simulink model "a2_pfc_rl"  (R2021b)
settings: Solver=FixedStepAuto  StartTime=0.0  StopTime=120  FixedStep=0.2  RelTol=1e-3
PreLoadFcn:
  | % Simulation parameters
  | %load exampleMap
InitFcn:
  | % paremeters of pure persuit
  | desired_v_robot_1=0.2
  | desired_w_robot_1=4
  | desired_lookahead_robot_1=0.2
  | 
  | % paremeters of recovery
  | recovery_w=0.5
  | 
  | sampleTime = 0.05;
  | 
  | % Robot parameters
  | wheelRadius = 0.025;
  | robotRadius = 0.15;
  | 
  | % Lidar parameters
  | sensorOffset = [0,0];
  | scanAngles = linspace(-pi/2,pi/2,9)';
  | maxRange = 5;
  | 
  | %%%%%%
  | ks=-1;
  | 
  | %初始位置
  | x_1_0=1;
  | y_1_0=0;
  | yaw_1_0=0.0;
  | 
  | x_2_0=0.6;
  | y_2_0=0;
  | yaw_2_0=0;
  | x_3_0=0;
  | y_3_0=0.6;
  | yaw_3_0=0;
  | 
  | x_4_0=0;
  | y_4_0=0.9;
  | yaw_4_0=0;
libraries: mobileRoboticsLib x3, simulink x2, robotmobilelib x2, robotalgslib x1, rllib x1
settings Model: Creator=scastro  LastModifiedBy=amov
settings SolverCC: ZeroCrossAlgorithm=Adaptive  AlgebraicLoopSolver=TrustRegion
settings DataIOCC: ReturnWorkspaceOutputs=off
settings OptimizationCC: EnhancedBackFolding=on  PassReuseOutputArgsAs=Individual arguments  ZeroExternalMemoryAtStartup=off  ZeroInternalMemoryAtStartup=off  MaxStackSize=64  OptimizeBlockOrder=speed  DifferentSizesBufferReuse=on  OptimizationCustomize=off  EfficientTunableParamExpr=on
settings DebuggingCC: ParameterTunabilityLossMsg=error  PregeneratedLibrarySubsystemCodeDiagnostic=none  SFMachineParentedDataDiag=warning  ArithmeticOperatorsInVariantConditions=warning
settings HardwareCC: ProdBitPerPointer=32  ProdBitPerSizeT=32  ProdBitPerPtrDiffT=32  ProdLargestAtomicFloat=None  ProdIntDivRoundTo=Undefined  ProdEndianess=Unspecified  ProdWordSize=32  ProdHWDeviceType=Generic->Unspecified (assume 32-bit Generic)
settings SFSimCC: SimUseLocalCustomCode=off  MATLABDynamicMemAlloc=off  CustomCodeUndefinedFunction=UseInterfaceOnly
settings RTWCC: Description=Embedded Coder  SystemTargetFile=ert.tlc  HardwareBoard=Robot Operating System (ROS)  TLCOptions="-aInlineSetEventsForThisBaseRateFcn=TLC_FALSE -aSuppressMultiTaskScheduler=TLC_FALSE  -aRateBasedStepFcn=0"  TemplateMakefile=ert_default_tmf  RTWUseLocalCustomCode=off  Toolchain=Catkin  TargetLang=C++
settings CodeAppCC: ForceParamTrailComments=on  IgnoreCustomStorageClasses=off  OperatorAnnotations=on  SimulinkDataObjDesc=on  SFDataObjDesc=on  InsertBlockDesc=on

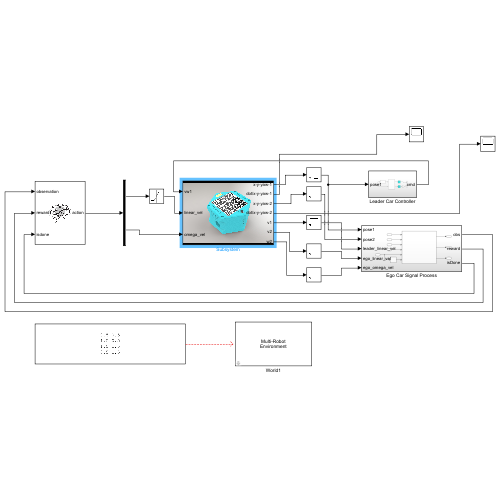
[thumbnail: Simulink's stored preview of the top-level diagram]
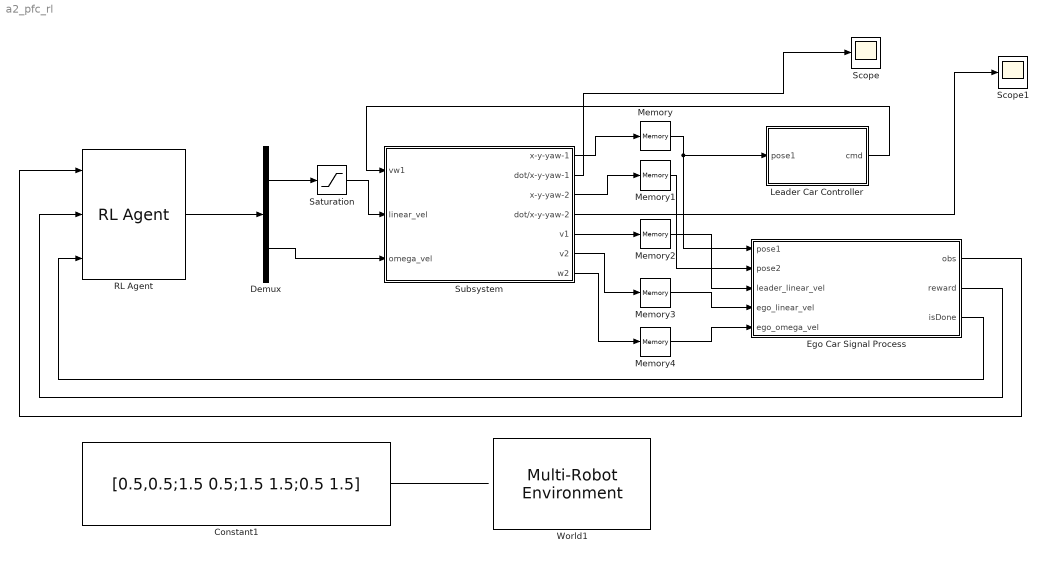
== system a2_pfc_rl ==
  Constant1 : Constant  Value=[0.5,0.5;1.5 0.5;1.5 1.5;0.5 1.5]
  Demux : Demux  Outputs=2
  Ego Car Signal Process : Subsystem
  Leader Car Controller : Subsystem
  Memory : Memory  InitialCondition=[x_1_0,y_1_0,yaw_1_0]
  Memory1 : Memory  InitialCondition=[x_2_0,y_2_0,yaw_2_0]
  Memory2 : Memory  InitialCondition=0.2
  Memory3 : Memory  InitialCondition=0.2
  Memory4 : Memory
  RL Agent : rllib/RL Agent  Agent=agent  ExternalActionAsInput=off  ProvideCumRwd=off  TreatAsDirectFeedthrough=on
  Saturation : Saturate  LowerLimit=0.1
  Scope : Scope
  Scope1 : Scope
  Subsystem : Subsystem
      mask Display: image('$imagefile'); % 使用工具条上的 "编辑图像" 进行更改。
  World1 : mobileRoboticsLib/Environments/Multi-Robot Environment  numRobots=2  showWaypoints=on  showObjects=off  objectColors=[1 0 0;0 1 0;0 0 1]  objectMarkers='s'  showRobotIds=on  plotSensorLines=on
      settings: SourceProductName=Mobile Robotics Simulation Toolbox
  wires:
  Subsystem/1(x-y-yaw-1) -> Memory/1
  Subsystem/3(x-y-yaw-2) -> Memory1/1
  Subsystem/5(v1) -> Memory2/1
  Subsystem/6(v2) -> Memory3/1
  Subsystem/7(w2) -> Memory4/1
  Memory1/1 -> Ego Car Signal Process/2(pose2)
  Memory2/1 -> Ego Car Signal Process/3(leader_linear_vel)
  Memory3/1 -> Ego Car Signal Process/4(ego_linear_vel)
  Memory4/1 -> Ego Car Signal Process/5(ego_omega_vel)
  Ego Car Signal Process/3(isDone) -> RL Agent/3
  Saturation/1 -> Subsystem/2(linear_vel)
  Demux/2 -> Subsystem/3(omega_vel)
  Subsystem/2(dot/x-y-yaw-1) -> Scope/1
  Subsystem/4(dot/x-y-yaw-2) -> Scope1/1
  Ego Car Signal Process/1(obs) -> RL Agent/1
  Ego Car Signal Process/2(reward) -> RL Agent/2
  RL Agent/1 -> Demux/1
  Demux/1 -> Saturation/1
  Memory/1 -> Ego Car Signal Process/1(pose1), Leader Car Controller/1(pose1)
  Leader Car Controller/1(cmd) -> Subsystem/1(vw1)
  Constant1/1 -> ?

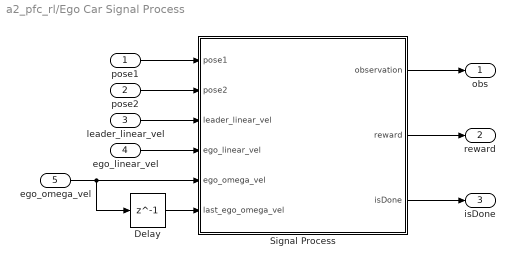
== system a2_pfc_rl/Ego Car Signal Process ==
  pose1 : Inport
  pose2 : Inport  Port=2
  leader_linear_vel : Inport  Port=3
  ego_linear_vel : Inport  Port=4
  ego_omega_vel : Inport  Port=5
  Delay : Delay  DelayLength=1  InitialCondition=0
  Signal Process : MATLAB Function  TreatAsAtomicUnit=on
  obs : Outport
  reward : Outport  Port=2
  isDone : Outport  Port=3
  wires:
  pose1/1 -> Signal Process/1(pose1)
  Signal Process/1(observation) -> obs/1
  leader_linear_vel/1 -> Signal Process/3(leader_linear_vel)
  Signal Process/3(isDone) -> isDone/1
  ego_omega_vel/1 -> Signal Process/5(ego_omega_vel), Delay/1
  pose2/1 -> Signal Process/2(pose2)
  ego_linear_vel/1 -> Signal Process/4(ego_linear_vel)
  Signal Process/2(reward) -> reward/1
  Delay/1 -> Signal Process/6(last_ego_omega_vel)

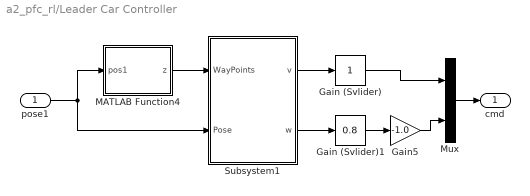
== system a2_pfc_rl/Leader Car Controller ==
  pose1 : Inport
  Gain (Svlider) : simulink/Math Operations/Slider Gain  gain=1  low=0.1  high=10
  Gain (Svlider)1 : simulink/Math Operations/Slider Gain  gain=0.8  low=0.1  high=3
  Gain5 : Gain  Gain=-1.0
  MATLAB Function4 : MATLAB Function  TreatAsAtomicUnit=on
  Mux : Mux  Inputs=2
  Subsystem1 : Subsystem
  cmd : Outport
  wires:
  Mux/1 -> cmd/1
  Subsystem1/1(v) -> Gain (Svlider)/1
  Gain (Svlider)/1 -> Mux/1
  pose1/1 -> Subsystem1/2(Pose), MATLAB Function4/1(pos1)
  Subsystem1/2(w) -> Gain (Svlider)1/1
  MATLAB Function4/1(z) -> Subsystem1/1(WayPoints)
  Gain (Svlider)1/1 -> Gain5/1
  Gain5/1 -> Mux/2

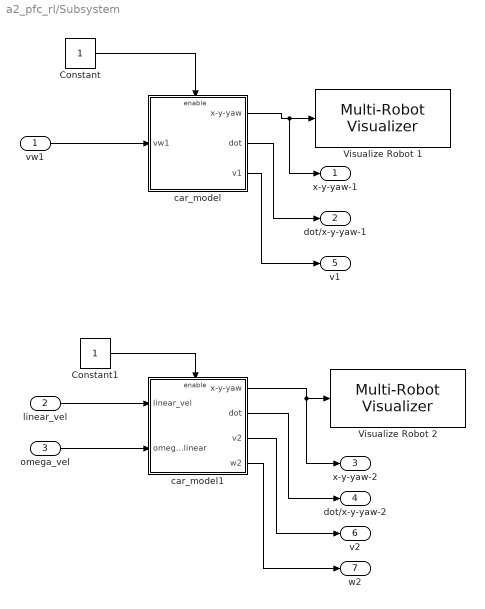
== system a2_pfc_rl/Subsystem ==
  vw1 : Inport
  linear_vel : Inport  Port=2
  omega_vel : Inport  Port=3
  Constant : Constant
  Constant1 : Constant
  Visualize Robot 1 : mobileRoboticsLib/Environments/Multi-Robot Visualizer  idx=1  radius=0.15  robotColor=[0 0 1]  showTraj=off  hasLidar=off  sensorOffset=sensorOffset  scanAngles=scanAngles  maxNumScans=0  hasObjDetector=off  objDetectorOffset=[0,0]  objDetectorAngle=0  objDetectorFOV=pi/2  objDetectorMaxRange=5  hasRobotDetector=off  robotDetectorOffset=[0,0]  robotDetectorAngle=0  robotDetectorFOV=pi/3  robotDetectorMaxRange=5  robotDetectorNumDetections=0
      settings: SourceProductName=Mobile Robotics Simulation Toolbox
  Visualize Robot 2 : mobileRoboticsLib/Environments/Multi-Robot Visualizer  idx=2  radius=0.15  robotColor=[1 0 0]  showTraj=on  hasLidar=off  sensorOffset=sensorOffset  scanAngles=scanAngles  maxNumScans=0  hasObjDetector=off  objDetectorOffset=[0 0]  objDetectorAngle=0  objDetectorFOV=pi/2  objDetectorMaxRange=5  hasRobotDetector=off  robotDetectorOffset=[0,0]  robotDetectorAngle=0  robotDetectorFOV=pi/3  robotDetectorMaxRange=5  robotDetectorNumDetections=0
      settings: SourceProductName=Mobile Robotics Simulation Toolbox
  car_model : Subsystem
  car_model1 : Subsystem
  x-y-yaw-1 : Outport
  dot/x-y-yaw-1 : Outport  Port=2
  x-y-yaw-2 : Outport  Port=3
  dot/x-y-yaw-2 : Outport  Port=4
  v1 : Outport  Port=5
  v2 : Outport  Port=6
  w2 : Outport  Port=7
  wires:
  Constant/1 -> car_model/Enable
  Constant1/1 -> car_model1/Enable
  car_model/1(x-y-yaw) -> x-y-yaw-1/1, Visualize Robot 1/1
  car_model1/1(x-y-yaw) -> x-y-yaw-2/1, Visualize Robot 2/1
  vw1/1 -> car_model/1(vw1)
  car_model/2(dot) -> dot/x-y-yaw-1/1
  car_model1/2(dot) -> dot/x-y-yaw-2/1
  car_model/3(v1) -> v1/1
  car_model1/3(v2) -> v2/1
  car_model1/4(w2) -> w2/1
  omega_vel/1 -> car_model1/2(omega_linear)
  linear_vel/1 -> car_model1/1(linear_vel)

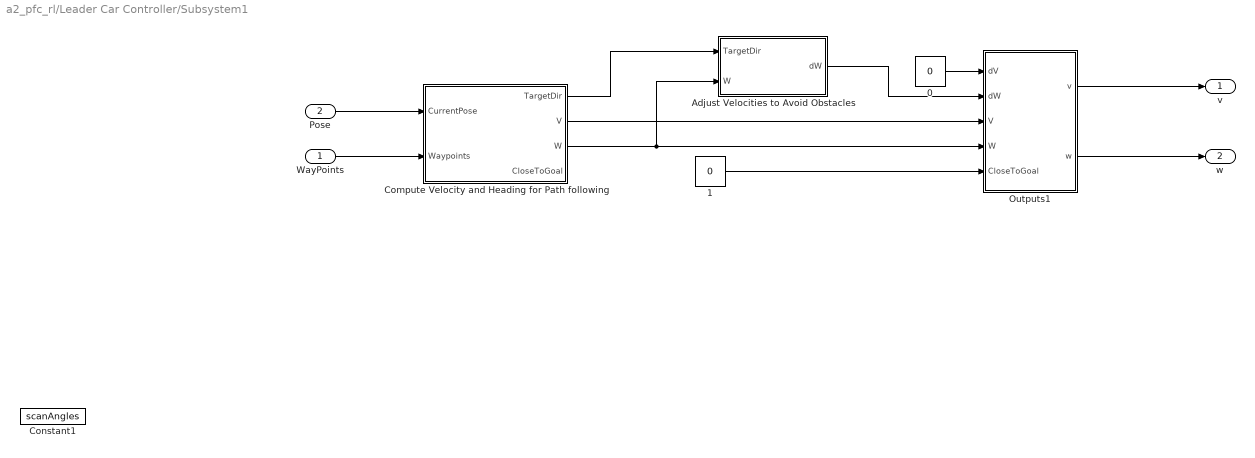
== system a2_pfc_rl/Leader Car Controller/Subsystem1 ==
  WayPoints : Inport
  Pose : Inport  Port=2
  0 : Constant  Value=0
  1 : Constant  Value=0
  Adjust Velocities to Avoid Obstacles : Subsystem
  Compute Velocity and Heading for Path following : Subsystem
  Constant1 : Constant  Value=scanAngles
  Outputs1 : Subsystem
  v : Outport
  w : Outport  Port=2
  wires:
  Compute Velocity and Heading for Path following/3(W) -> Adjust Velocities to Avoid Obstacles/2(W), Outputs1/4(W)
  Pose/1 -> Compute Velocity and Heading for Path following/1(CurrentPose)
  Compute Velocity and Heading for Path following/2(V) -> Outputs1/3(V)
  WayPoints/1 -> Compute Velocity and Heading for Path following/2(Waypoints)
  1/1 -> Outputs1/5(CloseToGoal)
  Outputs1/1(v) -> v/1
  Outputs1/2(w) -> w/1
  Adjust Velocities to Avoid Obstacles/1(dW) -> Outputs1/2(dW)
  0/1 -> Outputs1/1(dV)
  Compute Velocity and Heading for Path following/1(TargetDir) -> Adjust Velocities to Avoid Obstacles/1(TargetDir)

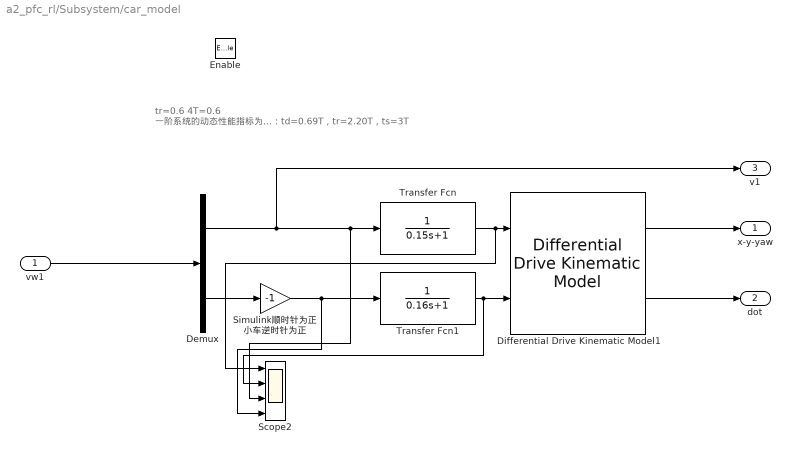
== system a2_pfc_rl/Subsystem/car_model ==
  note: tr=0.6
      | 4T=0.6
      | 一阶系统的动态性能指标为：td=0.69T，tr=2.20T，ts=3T
  vw1 : Inport
  Enable : EnablePort  ShowOutputPort=on
  Demux : Demux  Outputs=2
  Differential Drive Kinematic Model1 : robotmobilelib/Differential Drive Kinematic Model  VehicleInputs=Vehicle Speed & Heading Angular Velocity  WheelRadius=0.05  WheelSpeedRange=[-inf inf]  TrackWidth=0.2  InitialState=[x_1_0, y_1_0, yaw_1_0]'  SimulateUsing=Interpreted execution
      settings: SourceProductBaseCode=RO
  Scope2 : Scope  NumInputPorts=4
  Simulink顺时针为正 小车逆时针为正 : Gain  Gain=-1
  Transfer Fcn : TransferFcn  Denominator=[0.15 1]
  Transfer Fcn1 : TransferFcn  Denominator=[0.16 1]
  x-y-yaw : Outport
  dot : Outport  Port=2
  v1 : Outport  Port=3
  wires:
  Simulink顺时针为正 小车逆时针为正/1 -> Scope2/4, Transfer Fcn1/1
  Transfer Fcn/1 -> Differential Drive Kinematic Model1/1, Scope2/1
  Demux/1 -> Scope2/3, Transfer Fcn/1, v1/1
  Transfer Fcn1/1 -> Differential Drive Kinematic Model1/2, Scope2/2
  Demux/2 -> Simulink顺时针为正 小车逆时针为正/1
  vw1/1 -> Demux/1
  Differential Drive Kinematic Model1/1 -> x-y-yaw/1
  Differential Drive Kinematic Model1/2 -> dot/1

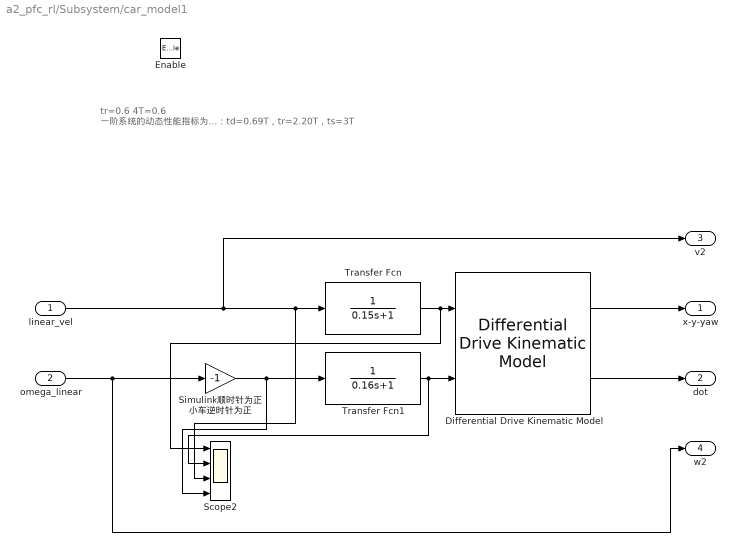
== system a2_pfc_rl/Subsystem/car_model1 ==
  note: tr=0.6
      | 4T=0.6
      | 一阶系统的动态性能指标为：td=0.69T，tr=2.20T，ts=3T
  linear_vel : Inport
  omega_linear : Inport  Port=2
  Enable : EnablePort  ShowOutputPort=on
  Differential Drive Kinematic Model : robotmobilelib/Differential Drive Kinematic Model  VehicleInputs=Vehicle Speed & Heading Angular Velocity  WheelRadius=0.05  WheelSpeedRange=[-inf inf]  TrackWidth=0.2  InitialState=[x_2_0, y_2_0, yaw_2_0]'  SimulateUsing=Interpreted execution
      settings: SourceProductBaseCode=RO
  Scope2 : Scope  NumInputPorts=4
  Simulink顺时针为正 小车逆时针为正 : Gain  Gain=-1
  Transfer Fcn : TransferFcn  Denominator=[0.15 1]
  Transfer Fcn1 : TransferFcn  Denominator=[0.16 1]
  x-y-yaw : Outport
  dot : Outport  Port=2
  v2 : Outport  Port=3
  w2 : Outport  Port=4
  wires:
  Simulink顺时针为正 小车逆时针为正/1 -> Scope2/4, Transfer Fcn1/1
  Transfer Fcn/1 -> Scope2/1, Differential Drive Kinematic Model/1
  linear_vel/1 -> v2/1, Scope2/3, Transfer Fcn/1
  Transfer Fcn1/1 -> Scope2/2, Differential Drive Kinematic Model/2
  Differential Drive Kinematic Model/1 -> x-y-yaw/1
  Differential Drive Kinematic Model/2 -> dot/1
  omega_linear/1 -> w2/1, Simulink顺时针为正 小车逆时针为正/1

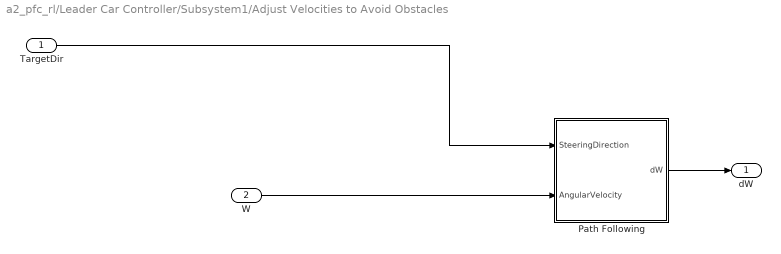
== system a2_pfc_rl/Leader Car Controller/Subsystem1/Adjust Velocities to Avoid Obstacles ==
  TargetDir : Inport
  W : Inport  Port=2
  Path Following : Subsystem  TreatAsAtomicUnit=on
  dW : Outport  VectorParamsAs1DForOutWhenUnconnected=off
  wires:
  Path Following/1(dW) -> dW/1
  W/1 -> Path Following/2(AngularVelocity)
  TargetDir/1 -> Path Following/1(SteeringDirection)

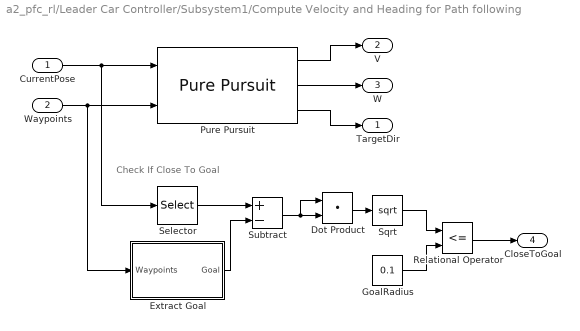
== system a2_pfc_rl/Leader Car Controller/Subsystem1/Compute Velocity and Heading for Path following ==
  note: Check If Close To Goal
  CurrentPose : Inport
  Waypoints : Inport  Port=2
  " Extract Goal" : MATLAB Function  TreatAsAtomicUnit=on
  Dot Product : DotProduct  InputSameDT=on  OutDataTypeStr=Inherit: Inherit via internal rule
  GoalRadius : Constant  Value=0.1
  Pure Pursuit : robotalgslib/Pure Pursuit  DesiredLinearVelocity=desired_v_robot_1  MaxAngularVelocity=desired_w_robot_1  LookaheadDistance=desired_lookahead_robot_1  TargetDirPort=on  SimulateUsing=Code generation
  Relational Operator : RelationalOperator  Operator=<=  OutDataTypeStr=boolean  RndMeth=Simplest
  Selector : Selector  InputPortWidth=3  IndexOptions=Index vector (dialog)  Indices=[1 2]  OutputSizes=1
  Sqrt : Sqrt  SaturateOnIntegerOverflow=on
  Subtract : Sum  Inputs=+-
  TargetDir : Outport  VectorParamsAs1DForOutWhenUnconnected=off
  V : Outport  Port=2  VectorParamsAs1DForOutWhenUnconnected=off
  W : Outport  Port=3  VectorParamsAs1DForOutWhenUnconnected=off
  CloseToGoal : Outport  Port=4  VectorParamsAs1DForOutWhenUnconnected=off
  wires:
  Pure Pursuit/3 -> TargetDir/1
  Pure Pursuit/2 -> W/1
  Pure Pursuit/1 -> V/1
  " Extract Goal"/1(Goal) -> Subtract/2
  Waypoints/1 -> " Extract Goal"/1(Waypoints), Pure Pursuit/2
  CurrentPose/1 -> Selector/1, Pure Pursuit/1
  Relational Operator/1 -> CloseToGoal/1
  GoalRadius/1 -> Relational Operator/2
  Selector/1 -> Subtract/1
  Dot Product/1 -> Sqrt/1
  Sqrt/1 -> Relational Operator/1
  Subtract/1 -> Dot Product/1, Dot Product/2

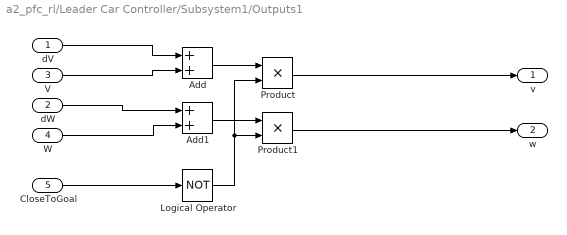
== system a2_pfc_rl/Leader Car Controller/Subsystem1/Outputs1 ==
  dV : Inport
  dW : Inport  Port=2
  V : Inport  Port=3
  W : Inport  Port=4
  CloseToGoal : Inport  Port=5
  Add : Sum
  Add1 : Sum
  Logical Operator : Logic  Operator=NOT  AllPortsSameDT=off  OutDataTypeStr=boolean
  Product : Product
  Product1 : Product
  v : Outport
  w : Outport  Port=2
  wires:
  V/1 -> Add/2
  W/1 -> Add1/2
  dV/1 -> Add/1
  dW/1 -> Add1/1
  CloseToGoal/1 -> Logical Operator/1
  Add/1 -> Product/1
  Add1/1 -> Product1/1
  Product1/1 -> w/1
  Product/1 -> v/1
  Logical Operator/1 -> Product1/2, Product/2

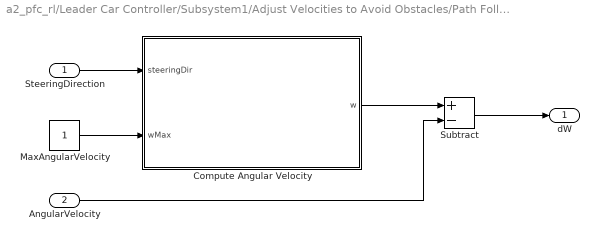
== system a2_pfc_rl/Leader Car Controller/Subsystem1/Adjust Velocities to Avoid Obstacles/Path Following ==
  SteeringDirection : Inport
  AngularVelocity : Inport  Port=2
  Compute Angular Velocity : MATLAB Function  TreatAsAtomicUnit=on
  MaxAngularVelocity : Constant
  Subtract : Sum  Inputs=+-
  dW : Outport  VectorParamsAs1DForOutWhenUnconnected=off
  wires:
  MaxAngularVelocity/1 -> Compute Angular Velocity/2(wMax)
  SteeringDirection/1 -> Compute Angular Velocity/1(steeringDir)
  Subtract/1 -> dW/1
  Compute Angular Velocity/1(w) -> Subtract/1
  AngularVelocity/1 -> Subtract/2

== matlab function a2_pfc_rl/Ego Car Signal Process/Signal Process ==
  data: observation output; reward output; isDone output; pose1 input; pose2 input; leader_linear_vel input size=1; ego_linear_vel input size=1; ego_omega_vel input size=1; last_ego_omega_vel input
function [observation, reward, isDone] = ...
    car2(pose1,pose2,leader_linear_vel, ego_linear_vel, ego_omega_vel, last_ego_omega_vel)


persistent sim_step  yaw_delta lateral_rel_dist

if isempty(sim_step)
    sim_step = 0;
end

if isempty(yaw_delta)
    yaw_delta = 0.0;
end

if isempty(lateral_rel_dist)
    lateral_rel_dist = 0.0;
end

x1=pose1(1);
y1=pose1(2);
yaw1=pose1(3);

x2=pose2(1);
y2=pose2(2);
yaw2=pose2(3);

observation = zeros(1,9);

isDone = 0;

yaw_delta_new = angdiff(yaw1, yaw2);

[rel_dist_new, lateral_rel_dist_new, longitudinal_rel_dist_new] = heng_zong_dist_calc(x1,y1,x2,y2, yaw1);

observation = get_obs(x1,x2,y1,y2,lateral_rel_dist_new, longitudinal_rel_dist_new, ...
    yaw_delta_new, leader_linear_vel, ego_linear_vel, yaw_delta, lateral_rel_dist);


isDone = EnvisDone(rel_dist_new, lateral_rel_dist_new, longitudinal_rel_dist_new);

e_v = observation(4);

reward = reward_calc(e_v, lateral_rel_dist_new, longitudinal_rel_dist_new, ego_linear_vel, ego_omega_vel, last_ego_omega_vel, isDone, sim_step);

sim_step = sim_step + 1;
yaw_delta = yaw_delta_new;
lateral_rel_dist = lateral_rel_dist_new;

end

function [rel_dist, heng_dist, zong_dist] = heng_zong_dist_calc(x1,y1,x2,y2, yaw1)

rel_yaw = atan2(y2-y1, x2-x1);

yaw_delta = angdiff(yaw1, rel_yaw);

rel_dist = sqrt(power(x2-x1,2.0)+power(y2-y1,2.0));

heng_dist = rel_dist*sin(yaw_delta);

zong_dist = rel_dist*cos(yaw_delta);

end

function v_ref = get_ref_velocity(leader_linear_vel, ego_linear_vel, longitudinal_rel_dist)
    t_gap = 1.0;
    D_default = 0.3;
    ego_v_set = 0.2;
    d_safe = ego_linear_vel * t_gap + D_default;

    if d_safe > longitudinal_rel_dist
        v_ref = min(leader_linear_vel, ego_v_set);
    else
        v_ref = ego_v_set;
    end
end

function observation = get_obs(x1,x2,y1,y2,lateral_rel_dist_new, longitudinal_rel_dist_new, ...
    yaw_delta_new, leader_linear_vel, ego_linear_vel, yaw_delta, lateral_rel_dist)  
    % 状态空间
    % longitudinal_rel_dist 前车与后车的纵向相对距离
    % lateral_rel_dist 前车与后车的横向相对距离
    % yaw_delta 前车与后车的航向角偏差
    % ego_linear_vel 后车的线速度
    % e_v 后车的参考速度与线速度之差
    % lateral_rel_dist_dot 前车与后车的横向相对距离变化率
    % yaw_delta_dot 前车与后车的航向角偏差变化率

    % 计算前车与后车的相对位置
    x_delta = x1 - x2;
    y_delta = y1 - y2;
    
    % 计算后车的横向偏移距离变化率和相对航向角变化率
    lateral_rel_dist_dot = lateral_rel_dist_new - lateral_rel_dist;
    yaw_delta_dot = yaw_delta_new - yaw_delta;

    % 计算后车的参考速度与线速度之差
    v_ref = get_ref_velocity(leader_linear_vel, ego_linear_vel, longitudinal_rel_dist_new);
    e_v = v_ref - ego_linear_vel;

    observation = [x_delta/2.0, y_delta/2.0, longitudinal_rel_dist_new/2.0, e_v/0.5, ego_linear_vel/0.5, ...
        lateral_rel_dist_new/2.0, lateral_rel_dist_dot/2.0, yaw_delta_new/pi, yaw_delta_dot/pi];
end

function flag = EnvisDone(rel_dist, lateral_rel_dist, longitudinal_rel_dist)
    flag = 0;
    avoid_dist = 0.18;

    max_lateral_rel_dist= 0.45;
    min_longitudinal_rel_dist = -0.5;

    if rel_dist <= avoid_dist
        flag = 1;
    end

    if longitudinal_rel_dist <= min_longitudinal_rel_dist || longitudinal_rel_dist >= 0
        flag = 1;
    end
    
    if abs(lateral_rel_dist) >= max_lateral_rel_dist
        flag = 1;
    end
end

function reward = reward_calc(e_v, lateral_rel_dist, longitudinal_rel_dist, ego_linear_vel, ego_omega_vel, last_ego_omega_vel, isDone, sim_step)
    F_t = 0.0;
    M_t = 0.0;
    H_t = 0.0;
    delta_omega = 0.0;
    
    e_v_square = e_v * e_v;
    lateral_rel_dist_square = lateral_rel_dist * lateral_rel_dist;
    longitudinal_rel_dist_square = longitudinal_rel_dist * longitudinal_rel_dist;

    if isDone==1
        F_t = 1.0;
    end

    if e_v_square < 1.0
        M_t = 1.0;
    end

    if lateral_rel_dist_square<0.01
        H_t = 1.0;
    end

    if sim_step >= 2
        delta_omega = ego_omega_vel - last_ego_omega_vel;
    end

    reward = -0.1*e_v_square - 0.1*ego_linear_vel*ego_linear_vel -0.3*lateral_rel_dist_square -0.3*longitudinal_rel_dist_square...
         - 0.5*ego_omega_vel*ego_omega_vel -0.4*delta_omega*delta_omega - 10.0*F_t + M_t + + 2.0*H_t;

end

== matlab function a2_pfc_rl/Leader Car Controller/Subsystem1/Adjust Velocities to Avoid Obstacles/Path Following/Compute Angular Velocity ==
  data: steeringDir input; w output; wMax input
function w = exampleHelperComputeAngularVelocity(steeringDir, wMax)
%EXAMPLEHELPERCOMPUTEANGULARVELOCITY Compute angular velocity
%   W = exampleHelperComputeAngularVelocity(STEERINGDIR)
%   returns the angular velocity W for a differential drive robot in radians
%   per second for a given steering direction STEERINGDIR in the robot's
%   coordinate frame in radians.
%
%   W = exampleHelperComputeAngularVelocity(STEERINGDIR, WMAX)
%   returns the angular velocity W for a differential drive robot in radians
%   per second for a given steering direction STEERINGDIR in the robot's
%   coordinate frame in radians and maximum angular velocity WMAX in
%   radians per second. The output angular velocity is saturated based on
%   the WMAX.
%
%   Example:
%       
%       w = exampleHelperComputeAngularVelocity(0.2, 1);

% Copyright 2015 The MathWorks, Inc.

%#codegen
%#ok<*EMCA>

% Allow variable input arguments
if nargin == 1   
    wMax = inf;
end

validateattributes(steeringDir, {'double'},{'real'},...
    'exampleHelperComputeAngularVelocity', 'STEERINGDIR', 1);
validateattributes(wMax, {'double'},{'real', 'positive'},...
    'exampleHelperComputeAngularVelocity', 'WMAX', 2);

% Computing in robot's coordinate frame
curPose = [0 0 0];

% The following computation is similar to robotics.PurePursuit
lookaheadPoint = [cos(steeringDir), sin(steeringDir)];
slope = atan2((lookaheadPoint(2) - curPose(2)), ...
    (lookaheadPoint(1) - curPose(1)));
alpha = angdiff(curPose(3), slope);

% Angular velocity command for a differential drive robot is
% equal to the desired curvature to be followed by the robot.

w = (2*sin(alpha));

% Pick a constant rotation when robot is facing in the opposite
% direction of the path
if abs(abs(alpha) - pi) < 1e-12
    w = sign(w)*1;
end

if abs(w) > wMax
    w = sign(w)*wMax;
end

end

== matlab function a2_pfc_rl/Leader Car Controller/Subsystem1/Compute Velocity and Heading for Path following/ Extract Goal ==
  data: Waypoints input; Goal output
function Goal = extractGoal(Waypoints)
%#codegen
b = isnan(Waypoints);
[rows,~] = find(b);
ridx = setdiff(1:size(Waypoints,1), sort(rows));
Goal = [Waypoints(ridx(end), 1) Waypoints(ridx(end), 2)];

== matlab function a2_pfc_rl/Leader Car Controller/MATLAB Function4 ==
  data: z output; pos1 input
function z = plot_a_square(pos1)
% 
% persistent Waypoints idx
% if isempty(Waypoints)
%     Waypoints=[0.2,0.2;1.8 0.2;1.8 1.8;0.2 1.8];
%     idx=0;
% end
% if idx==0
%     %初始化
%     [~,idx]=max([norm(Waypoints(1,:)-pos1(1:2)'),norm(Waypoints(2,:)-pos1(1:2)'),norm(Waypoints(3,:)-pos1(1:2)'),norm(Waypoints(4,:)-pos1(1:2)')]);
% end
% 
% if norm([Waypoints(idx,:)-pos1(1:2)'])<0.25
%     idx=idx+1;
%     if idx>length(Waypoints(:,1))
%         idx=1;
%     end
% end
% z=Waypoints(idx,:);


persistent Waypoints idx

if isempty(Waypoints)
    Waypoints=[0.5,0.5;1.5 0.5;1.5 1.5;0.5 1.5];
    idx=2;
end

if idx == 4
    pre_waypt = Waypoints(4-1,:)';
    curr_waypt = Waypoints(idx,:)';
    next_waypt = Waypoints(1,:)';
else
    if idx == 1
        pre_waypt = Waypoints(4,:)';
        curr_waypt = Waypoints(1,:)';
        next_waypt = Waypoints(2,:)';
    else
        pre_waypt = Waypoints(idx-1,:)';
        curr_waypt = Waypoints(idx,:)';
        next_waypt = Waypoints(idx+1,:)';
    end
end

pre_q = vec_norm(curr_waypt, pre_waypt);
next_q = vec_norm(next_waypt, curr_waypt);

curr_n = vec_normalize(pre_q + next_q);
curr_diff = vec_norm(pos1(1:2), curr_waypt);

flag = dot(curr_diff, curr_n);

if flag >=0

    if idx < 4
        idx = idx + 1;
    else
        idx = 1;
    end
end

idx
z=Waypoints(idx,:)

end

function result = vec_normalize(vec)
    mag = vec_mag(vec);

    if mag>0
        result = vec * (1.0/mag);
    else
        result = [0.0, 0.0];
    end
end

function result = vec_norm(vec1, vec2)
    result = vec1 - vec2;
    result = vec_normalize(result);
end

function result = vec_mag(vec)
    result = sqrt(vec(1)*vec(1)+ vec(2)*vec(2));
end
